simulink model "Laborversuch_2_b"  (R2023b)
settings: Solver=VariableStepAuto  StartTime=0.0  StopTime=40  MaxStep=0.001  RelTol=1e-3
values from neighbouring files (symbols this model uses):
  AB = 0.0226    [Versuch_2_parameter_c.m]
  C = 0.003    [Versuch_2_parameter_c.m]
  KR = 0.01    [Versuch_2_parameter_c.m]
  TN = TN_array(count)    [Versuch_2_parameter_c.m]
settings Model: Creator=danie  LastModifiedBy=danie

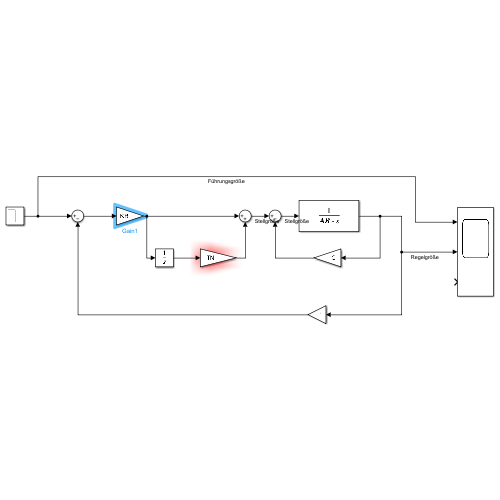
[thumbnail: Simulink's stored preview of the top-level diagram]
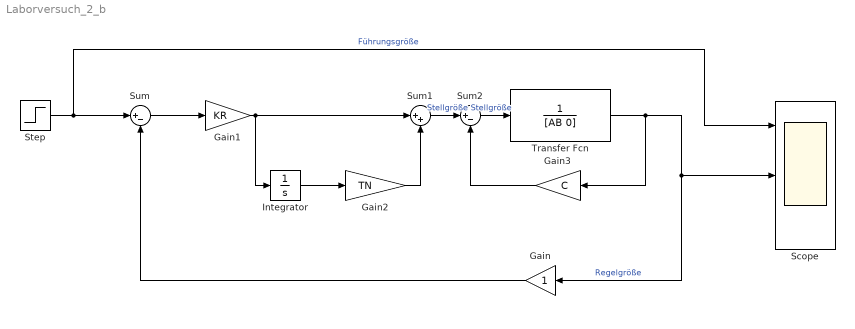
== system Laborversuch_2_b ==
  Gain : Gain
  Gain1 : Gain  Gain=KR
  Gain2 : Gain  Gain=TN
  Gain3 : Gain  Gain=C
  Integrator : Integrator
  Scope : Scope  NumInputPorts=3
  Step : Step  Time=100  Before=0.1  After=0  SampleTime=0
  Sum : Sum  Inputs=|+-
  Sum1 : Sum  Inputs=|++
  Sum2 : Sum  Inputs=|+-
  Transfer Fcn : TransferFcn  Denominator=[AB 0]
  wires:
  Transfer Fcn/1 -> Gain3/1, Scope/2, Gain/1  "Regelgröße"
  Gain/1 -> Sum/2
  Step/1 -> Sum/1, Scope/1  "Führungsgröße"
  Gain2/1 -> Sum1/2
  Gain1/1 -> Integrator/1, Sum1/1
  Sum/1 -> Gain1/1
  Integrator/1 -> Gain2/1
  Sum2/1 -> Transfer Fcn/1  "Stellgröße"
  Sum1/1 -> Sum2/1  "Stellgröße"
  Gain3/1 -> Sum2/2
